simulink model "e1"  (R2019b)
settings: Solver=FixedStepAuto  StartTime=0.0  StopTime=5  FixedStep=0.001  RelTol=1e-3
settings Model: Creator=12603  LastModifiedBy=12603
settings SolverCC: MaxConsecutiveMinStep=0.001

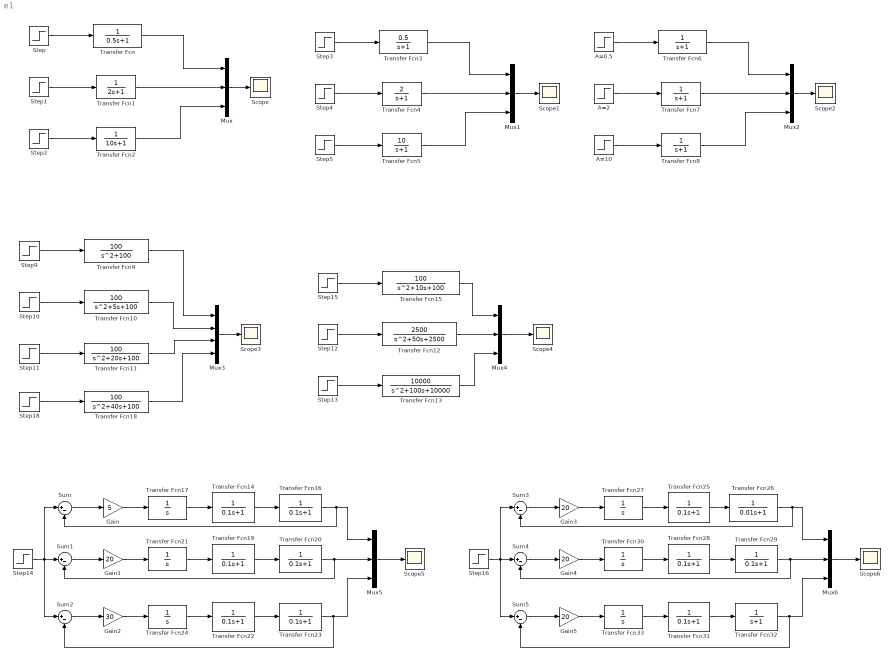
== system e1 ==
  A=0.5 : Step  Time=0  After=0.5  SampleTime=0
  A=10 : Step  Time=0  After=10  SampleTime=0
  A=2 : Step  Time=0  After=2  SampleTime=0
  Gain : Gain  Gain=5
  Gain{1,3..5} (4 alike) : Gain  Gain=20
  Gain2 : Gain  Gain=30
  Mux{,1..2,4..6} (6 alike) : Mux  Inputs=3
  Mux3 : Mux
  Scope{,1..6} (7 alike) : Scope
  Step{,1..5,9..16,18} (15 alike) : Step  Time=0  SampleTime=0
  Sum{,1..5} (6 alike) : Sum  Inputs=|+-
  Transfer Fcn : TransferFcn  Denominator=[0.5 1]
  Transfer Fcn1 : TransferFcn  Denominator=[2 1]
  Transfer Fcn10 : TransferFcn  Numerator=[100]  Denominator=[1 5 100]
  Transfer Fcn11 : TransferFcn  Numerator=[100]  Denominator=[1 20 100]
  Transfer Fcn12 : TransferFcn  Numerator=[2500]  Denominator=[1 50 2500]
  Transfer Fcn13 : TransferFcn  Numerator=[10000]  Denominator=[1 100 10000]
  Transfer Fcn{14,16,19..20,22..23,25,28..29,31} (10 alike) : TransferFcn  Denominator=[0.1 1]
  Transfer Fcn15 : TransferFcn  Numerator=[100]  Denominator=[1 10 100]
  Transfer Fcn{17,21,24,27,30,33} (6 alike) : TransferFcn  Denominator=[1 0]
  Transfer Fcn18 : TransferFcn  Numerator=[100]  Denominator=[1 40 100]
  Transfer Fcn2 : TransferFcn  Denominator=[10 1]
  Transfer Fcn26 : TransferFcn  Denominator=[0.01 1]
  Transfer Fcn3 : TransferFcn  Numerator=[0.5]  Denominator=[1 1]
  Transfer Fcn{6..8,32} (4 alike) : TransferFcn  Denominator=[1 1]
  Transfer Fcn4 : TransferFcn  Numerator=[2]  Denominator=[1 1]
  Transfer Fcn5 : TransferFcn  Numerator=[10]  Denominator=[1 1]
  Transfer Fcn9 : TransferFcn  Numerator=[100]  Denominator=[1 0 100]
  wires:
  Step2/1 -> Transfer Fcn2/1
  Mux/1 -> Scope/1
  Step3/1 -> Transfer Fcn3/1
  Mux1/1 -> Scope1/1
  Mux2/1 -> Scope2/1
  Step/1 -> Transfer Fcn/1
  Step1/1 -> Transfer Fcn1/1
  Transfer Fcn1/1 -> Mux/2
  Transfer Fcn/1 -> Mux/1
  Transfer Fcn2/1 -> Mux/3
  Step4/1 -> Transfer Fcn4/1
  Step5/1 -> Transfer Fcn5/1
  Transfer Fcn4/1 -> Mux1/2
  Transfer Fcn3/1 -> Mux1/1
  Transfer Fcn5/1 -> Mux1/3
  A=0.5/1 -> Transfer Fcn6/1
  A=2/1 -> Transfer Fcn7/1
  A=10/1 -> Transfer Fcn8/1
  Transfer Fcn7/1 -> Mux2/2
  Transfer Fcn6/1 -> Mux2/1
  Transfer Fcn8/1 -> Mux2/3
  Step10/1 -> Transfer Fcn10/1
  Step11/1 -> Transfer Fcn11/1
  Step9/1 -> Transfer Fcn9/1
  Transfer Fcn9/1 -> Mux3/1
  Transfer Fcn10/1 -> Mux3/2
  Transfer Fcn11/1 -> Mux3/3
  Mux3/1 -> Scope3/1
  Step18/1 -> Transfer Fcn18/1
  Transfer Fcn18/1 -> Mux3/4
  Step15/1 -> Transfer Fcn15/1
  Step13/1 -> Transfer Fcn13/1
  Step12/1 -> Transfer Fcn12/1
  Transfer Fcn12/1 -> Mux4/2
  Transfer Fcn15/1 -> Mux4/1
  Transfer Fcn13/1 -> Mux4/3
  Mux4/1 -> Scope4/1
  Transfer Fcn14/1 -> Transfer Fcn16/1
  Step14/1 -> Sum/1, Sum2/1, Sum1/1
  Transfer Fcn17/1 -> Transfer Fcn14/1
  Transfer Fcn19/1 -> Transfer Fcn20/1
  Transfer Fcn22/1 -> Transfer Fcn23/1
  Transfer Fcn24/1 -> Transfer Fcn22/1
  Transfer Fcn21/1 -> Transfer Fcn19/1
  Transfer Fcn20/1 -> Sum1/2, Mux5/2
  Transfer Fcn16/1 -> Sum/2, Mux5/1
  Transfer Fcn23/1 -> Sum2/2, Mux5/3
  Gain/1 -> Transfer Fcn17/1
  Sum/1 -> Gain/1
  Gain1/1 -> Transfer Fcn21/1
  Sum1/1 -> Gain1/1
  Gain2/1 -> Transfer Fcn24/1
  Sum2/1 -> Gain2/1
  Mux5/1 -> Scope5/1
  Sum3/1 -> Gain3/1
  Gain4/1 -> Transfer Fcn30/1
  Gain3/1 -> Transfer Fcn27/1
  Transfer Fcn32/1 -> Sum5/2, Mux6/3
  Sum5/1 -> Gain5/1
  Transfer Fcn29/1 -> Sum4/2, Mux6/2
  Transfer Fcn26/1 -> Sum3/2, Mux6/1
  Gain5/1 -> Transfer Fcn33/1
  Transfer Fcn31/1 -> Transfer Fcn32/1
  Transfer Fcn33/1 -> Transfer Fcn31/1
  Transfer Fcn30/1 -> Transfer Fcn28/1
  Step16/1 -> Sum3/1, Sum5/1, Sum4/1
  Transfer Fcn28/1 -> Transfer Fcn29/1
  Transfer Fcn25/1 -> Transfer Fcn26/1
  Sum4/1 -> Gain4/1
  Mux6/1 -> Scope6/1
  Transfer Fcn27/1 -> Transfer Fcn25/1
